simulink library "acparams_lib"  (Simulink 7.2)
settings: Solver=ode45  SolverMode=SingleTasking  StartTime=0.0  StopTime=10.0  RelTol=1e-3
undefined symbols (not defined in the file or in its folder): aftfuel, aftfuel_pos, b, Cbar, cg_pos0, cg_shift_gear, DamageCase, DamageModels, DamageOnsetTime, engl_pos, engr_pos, fwdfuel, fwdfuel_pos, Inertia0, Inertia_shift_gear, ref_cg, S, w0
libraries: aeroutilslib x3, simulink x1
settings Model: Creator=amurch  LastModifiedBy=amurch  ExtModeAutoUpdateStatusClock=off

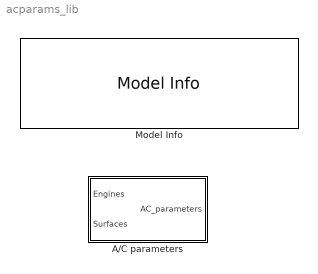
== system acparams_lib ==
  A/C parameters : Subsystem
  Model Info : simulink/Model-Wide Utilities/Model Info  SystemSampleTime=-1  InitialBlockCM=None  BlockCM=None  Frame=on  DisplayStringWithTags=|  HorizontalTextAlignment=Center  LeftAlignmentValue=0.5  SourceBlockDiagram=acparams_lib  TagMaxNumber=20
      | Aircraft Parameters Library
      | %<ModelVersion>
      | Las modified by %<LastModifiedBy> on %<LastModificationDate>

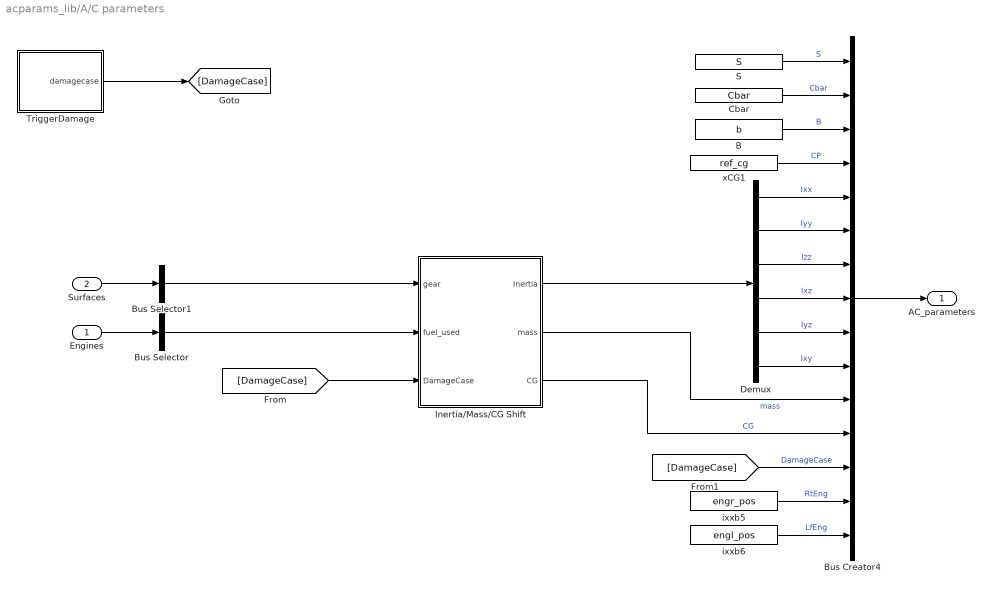
== system acparams_lib/A/C parameters ==
  Engines : Inport  OutDataType=sfix(16)  OutScaling=2^0
  Surfaces : Inport  Port=2  OutDataType=sfix(16)  OutScaling=2^0
  B : Constant  Value=b  OutDataType=sfix(16)  OutScaling=2^0
  Bus Creator4 : BusCreator  Inputs=15
  Bus Selector : BusSelector  OutputSignals=fuel_used
  Bus Selector1 : BusSelector  OutputSignals=GEAR
  Cbar : Constant  Value=Cbar  OutDataType=sfix(16)  OutScaling=2^0
  Demux : Demux  Outputs=6
  Inertia/Mass/CG Shift : Subsystem  mask{DamageModels=DamageModels}
      mask prompts: DamageModels "Array of Damage Cases"
      mask init:
      | Ncases=length(DamageModels);
      | dCGDamage=zeros(Ncases+1,3);   
      | dMassDamage=zeros(Ncases+1,1);
      | dInertiaDamage=zeros(Ncases+1,6);
      | for i=1:Ncases,
      |   if isfield(DamageModels{i},'Mass'),
      |      dInertiaDamage(i+1,:)=DamageModels{i}.Mass.dIxxIyyIzzIxzIyzIxy;
      |      dCGDamage(i+1,:)=DamageModels{i}.Mass.dCG;
      |      dMassDamage(i+1)=DamageModels{i}.Mass.dWeight;
      |   end
      | end
  S : Constant  Value=S  OutDataType=sfix(16)  OutScaling=2^0
  TriggerDamage : Subsystem
  ixxb5 : Constant  Value=engr_pos  OutDataType=sfix(16)  OutScaling=2^0
  ixxb6 : Constant  Value=engl_pos  OutDataType=sfix(16)  OutScaling=2^0
  xCG1 : Constant  Value=ref_cg  OutDataType=sfix(16)  OutScaling=2^0
  AC_parameters : Outport  OutDataType=sfix(16)  OutScaling=2^0
  wires:
  Bus Creator4/1 -> AC_parameters/1
  Engines/1 -> Bus Selector/1
  Surfaces/1 -> Bus Selector1/1
  Inertia/Mass/CG Shift/1(Inertia) -> Demux/1
  TriggerDamage/1(damagecase) -> [DamageCase]
  S/1 -> Bus Creator4/1  "S"
  Cbar/1 -> Bus Creator4/2  "Cbar"
  B/1 -> Bus Creator4/3  "B"
  xCG1/1 -> Bus Creator4/4  "CP"
  ixxb5/1 -> Bus Creator4/14  "RtEng"
  ixxb6/1 -> Bus Creator4/15  "LfEng"
  Demux/1 -> Bus Creator4/5  "Ixx"
  Demux/2 -> Bus Creator4/6  "Iyy"
  Demux/3 -> Bus Creator4/7  "Izz"
  Demux/4 -> Bus Creator4/8  "Ixz"
  Demux/5 -> Bus Creator4/9  "Iyz"
  Demux/6 -> Bus Creator4/10  "Ixy"
  Inertia/Mass/CG Shift/2(mass) -> Bus Creator4/11  "mass"
  Inertia/Mass/CG Shift/3(CG) -> Bus Creator4/12  "CG"
  [DamageCase] -> Bus Creator4/13  "DamageCase"
  [DamageCase] -> Inertia/Mass/CG Shift/3(DamageCase)
  Bus Selector1/1 -> Inertia/Mass/CG Shift/1(gear)
  Bus Selector/1 -> Inertia/Mass/CG Shift/2(fuel_used)

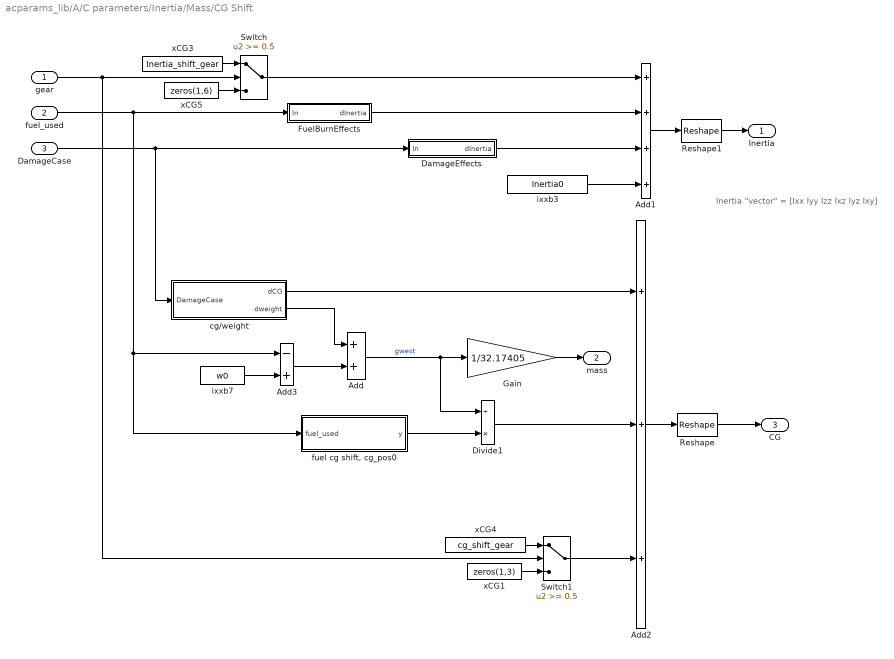
== system acparams_lib/A/C parameters/Inertia/Mass/CG Shift ==
  note: Inertia "vector" = [Ixx Iyy Izz Ixz Iyz Ixy]
  gear : Inport  OutDataType=sfix(16)  OutScaling=2^0
  fuel_used : Inport  Port=2  OutDataType=sfix(16)  OutScaling=2^0
  DamageCase : Inport  Port=3  OutDataType=sfix(16)  OutScaling=2^0
  Add : Sum  OutDataType=sfix(16)  OutScaling=2^-10
  Add1 : Sum  Inputs=++++  OutDataType=sfix(16)  OutScaling=2^-10
  Add2 : Sum  Inputs=+++  OutDataType=sfix(16)  OutScaling=2^-10
  Add3 : Sum  Inputs=-+  OutDataType=sfix(16)  OutScaling=2^-10
  DamageEffects : Subsystem
  Divide1 : Product  Inputs=/*  OutDataType=sfix(16)  OutScaling=2^-10
  FuelBurnEffects : Subsystem
  Gain : Gain  Gain=1/32.17405  ParameterDataType=sfix(16)  ParameterScaling=2^0  OutDataType=sfix(16)  OutScaling=2^0
  Reshape : Reshape
  Reshape1 : Reshape
  Switch : Switch  Threshold=0.5
  Switch1 : Switch  Threshold=0.5
  cg/weight : Subsystem
  "fuel cg shift, cg_pos0" : Stateflow chart
  ixxb3 : Constant  Value=Inertia0  OutDataType=sfix(16)  OutScaling=2^0
  ixxb7 : Constant  Value=w0  OutDataType=sfix(16)  OutScaling=2^0
  xCG1 : Constant  Value=zeros(1,3)  OutDataType=sfix(16)  OutScaling=2^0
  xCG3 : Constant  Value=Inertia_shift_gear  OutDataType=sfix(16)  OutScaling=2^0
  xCG4 : Constant  Value=cg_shift_gear  OutDataType=sfix(16)  OutScaling=2^0
  xCG5 : Constant  Value=zeros(1,6)  OutDataType=sfix(16)  OutScaling=2^0
  Inertia : Outport  OutDataType=sfix(16)  OutScaling=2^0
  mass : Outport  Port=2  OutDataType=sfix(16)  OutScaling=2^0
  CG : Outport  Port=3  OutDataType=sfix(16)  OutScaling=2^0
  wires:
  FuelBurnEffects/1(dInertia) -> Add1/2
  Switch/1 -> Add1/1
  Add1/1 -> Reshape1/1
  xCG3/1 -> Switch/1
  xCG5/1 -> Switch/3
  fuel_used/1 -> FuelBurnEffects/1(In), Add3/1, "fuel cg shift, cg_pos0"/1(fuel_used)
  ixxb3/1 -> Add1/4
  DamageEffects/1(dInertia) -> Add1/3
  DamageCase/1 -> DamageEffects/1(In), cg/weight/1(DamageCase)
  Add/1 -> Gain/1, Divide1/1  "gwest"
  Add2/1 -> Reshape/1
  Gain/1 -> mass/1
  ixxb7/1 -> Add3/2
  Switch1/1 -> Add2/3
  xCG4/1 -> Switch1/1
  xCG1/1 -> Switch1/3
  Add3/1 -> Add/2
  cg/weight/1(dCG) -> Add2/1
  gear/1 -> Switch/2, Switch1/2
  cg/weight/2(dweight) -> Add/1
  Reshape/1 -> CG/1
  Reshape1/1 -> Inertia/1
  Divide1/1 -> Add2/2
  "fuel cg shift, cg_pos0"/1(y) -> Divide1/2

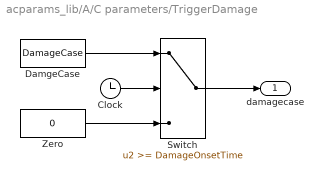
== system acparams_lib/A/C parameters/TriggerDamage ==
  Clock : Clock
      settings: Decimation=10
  DamgeCase : Constant  Value=DamageCase  OutDataType=sfix(16)  OutScaling=2^0
  Switch : Switch  Threshold=DamageOnsetTime
  Zero : Constant  Value=0  OutDataType=sfix(16)  OutScaling=2^0
  damagecase : Outport  OutDataType=sfix(16)  OutScaling=2^0
  wires:
  DamgeCase/1 -> Switch/1
  Zero/1 -> Switch/3
  Switch/1 -> damagecase/1
  Clock/1 -> Switch/2

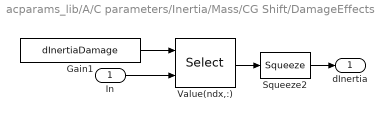
== system acparams_lib/A/C parameters/Inertia/Mass/CG Shift/DamageEffects ==
  In : Inport  OutDataType=sfix(16)  OutScaling=2^0
  Gain1 : Constant  Value=dInertiaDamage  OutDataType=sfix(16)  OutScaling=2^0
  Squeeze2 : Squeeze
  Value(ndx,:) : Selector  NumberOfDimensions=2  IndexMode=Zero-based  InputPortWidth=3  IndexOptions=Index vector (port),Select all  Indices=[1 3],1  OutputSizes=1,1
  dInertia : Outport  OutDataType=sfix(16)  OutScaling=2^0
  wires:
  In/1 -> Value(ndx,:)/2
  Gain1/1 -> Value(ndx,:)/1
  Value(ndx,:)/1 -> Squeeze2/1
  Squeeze2/1 -> dInertia/1

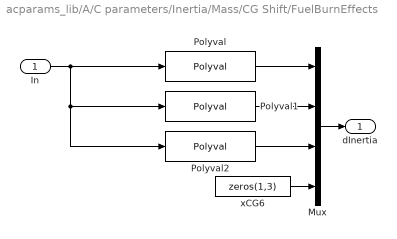
== system acparams_lib/A/C parameters/Inertia/Mass/CG Shift/FuelBurnEffects ==
  In : Inport  OutDataType=sfix(16)  OutScaling=2^0
  Mux : Mux
  Polyval : aeroutilslib/Polyval  SystemSampleTime=-1  p=Ixx_model
  Polyval1 : aeroutilslib/Polyval  SystemSampleTime=-1  p=Iyy_model
  Polyval2 : aeroutilslib/Polyval  SystemSampleTime=-1  p=Izz_model
  xCG6 : Constant  Value=zeros(1,3)  OutDataType=sfix(16)  OutScaling=2^0
  dInertia : Outport  OutDataType=sfix(16)  OutScaling=2^0
  wires:
  In/1 -> Polyval/1, Polyval1/1, Polyval2/1
  xCG6/1 -> Mux/4
  Polyval/1 -> Mux/1
  Polyval1/1 -> Mux/2
  Polyval2/1 -> Mux/3
  Mux/1 -> dInertia/1

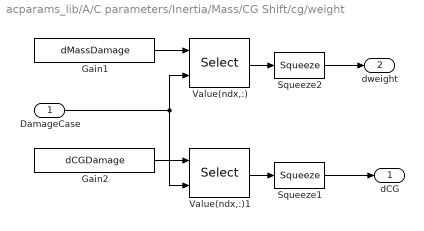
== system acparams_lib/A/C parameters/Inertia/Mass/CG Shift/cg/weight ==
  DamageCase : Inport  OutDataType=sfix(16)  OutScaling=2^0
  Gain1 : Constant  Value=dMassDamage  OutDataType=sfix(16)  OutScaling=2^0
  Gain2 : Constant  Value=dCGDamage  OutDataType=sfix(16)  OutScaling=2^0
  Squeeze1 : Squeeze
  Squeeze2 : Squeeze
  Value(ndx,:) : Selector  IndexMode=Zero-based  IndexOptions=Index vector (port)  Indices=[1 3]  OutputSizes=1
  Value(ndx,:)1 : Selector  NumberOfDimensions=2  IndexMode=Zero-based  InputPortWidth=3  IndexOptions=Index vector (port),Select all  Indices=[1 3],1  OutputSizes=1,1
  dCG : Outport  OutDataType=sfix(16)  OutScaling=2^0
  dweight : Outport  Port=2  OutDataType=sfix(16)  OutScaling=2^0
  wires:
  Gain2/1 -> Value(ndx,:)1/1
  Value(ndx,:)1/1 -> Squeeze1/1
  DamageCase/1 -> Value(ndx,:)/2, Value(ndx,:)1/2
  Gain1/1 -> Value(ndx,:)/1
  Value(ndx,:)/1 -> Squeeze2/1
  Squeeze1/1 -> dCG/1
  Squeeze2/1 -> dweight/1

== matlab function A/C parameters/Inertia/Mass/CG Shift/fuel cg shift, cg_pos0 ==
  data: fuel_used input double; y output double; aftfuel parameter double; fwdfuel parameter double; aftfuel_pos parameter double; fwdfuel_pos parameter double; w0 parameter double; cg_pos0 parameter double
function y = fcn(fuel_used,aftfuel,fwdfuel,aftfuel_pos,fwdfuel_pos,w0,cg_pos0)
% This block supports an embeddable subset of the MATLAB language.
% See the help menu for details. 

y = w0.*cg_pos0 - min(aftfuel,fuel_used).*aftfuel_pos - max(0,fuel_used-fwdfuel).*fwdfuel_pos;
